simulink model "HX_2023b_mdl"  (R2023b)
settings: Solver=ode4  StartTime=0  StopTime=300  FixedStep=0.01  RelTol=1e-3
undefined symbols (not defined in the file): f11, f22, g11_a, g11_b, g12_a, g21_a, g22_a, g22_b, P0
settings Model: SimulationMode=accelerator  Creator=mohammadodeh  LastModifiedBy=mohammadodeh

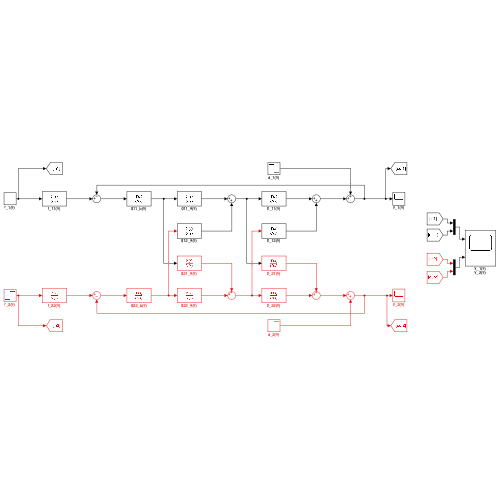
[thumbnail: Simulink's stored preview of the top-level diagram]
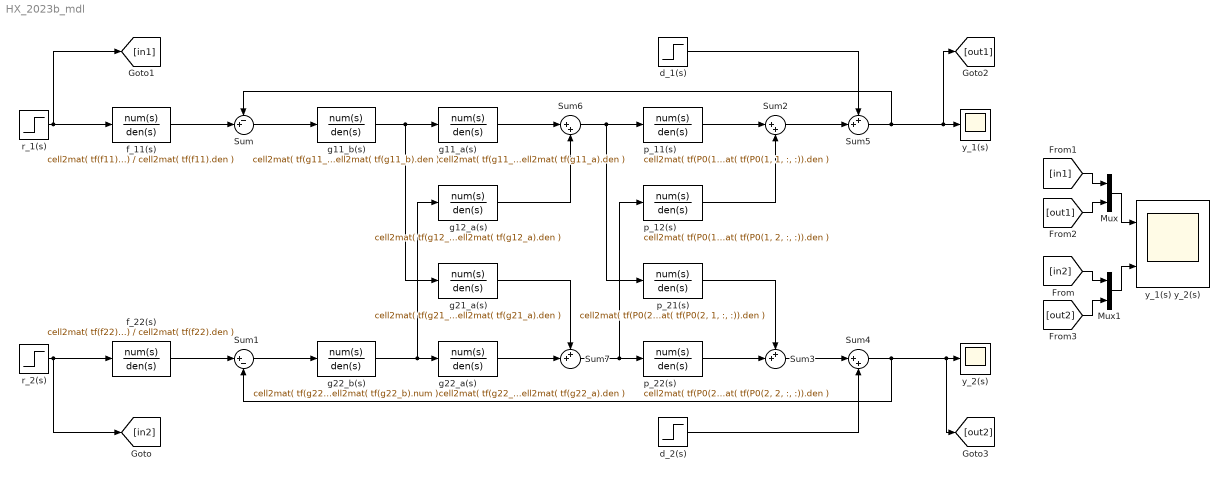
== system HX_2023b_mdl ==
  Mux : Mux  Inputs=2
  Mux1 : Mux  Inputs=2
  Sum : Sum  Inputs=-+|
  Sum1 : Sum  Inputs=|+-
  Sum2 : Sum  Inputs=|++
  Sum3 : Sum  Inputs=++|
  Sum4 : Sum  Inputs=|++
  Sum5 : Sum  Inputs=++|
  Sum6 : Sum  Inputs=|++
  Sum7 : Sum  Inputs=++|
  d_1(s) : Step  Time=250  After=-1  SampleTime=0
  d_2(s) : Step  Time=120  After=0.25  SampleTime=0
  f_11(s) : TransferFcn  Numerator=cell2mat( tf(f11).num )  Denominator=cell2mat( tf(f11).den )
  f_22(s) : TransferFcn  Numerator=cell2mat( tf(f22).num )  Denominator=cell2mat( tf(f22).den )
  g11_a(s) : TransferFcn  Numerator=cell2mat( tf(g11_a).num )  Denominator=cell2mat( tf(g11_a).den )
  g11_b(s) : TransferFcn  Numerator=cell2mat( tf(g11_b).num )  Denominator=cell2mat( tf(g11_b).den )
  g12_a(s) : TransferFcn  Numerator=cell2mat( tf(g12_a).num )  Denominator=cell2mat( tf(g12_a).den )
  g21_a(s) : TransferFcn  Numerator=cell2mat( tf(g21_a).num )  Denominator=cell2mat( tf(g21_a).den )
  g22_a(s) : TransferFcn  Numerator=cell2mat( tf(g22_a).num )  Denominator=cell2mat( tf(g22_a).den )
  g22_b(s) : TransferFcn  Numerator=cell2mat( tf(g22_b).num )  Denominator=cell2mat( tf(g22_b).num )
  p_11(s) : TransferFcn  Numerator=cell2mat( tf(P0(1, 1, :, :)).num )  Denominator=cell2mat( tf(P0(1, 1, :, :)).den )
  p_12(s) : TransferFcn  Numerator=cell2mat( tf(P0(1, 2, :, :)).num )  Denominator=cell2mat( tf(P0(1, 2, :, :)).den )
  p_21(s) : TransferFcn  Numerator=cell2mat( tf(P0(2, 1, :, :)).num )  Denominator=cell2mat( tf(P0(2, 1, :, :)).den )
  p_22(s) : TransferFcn  Numerator=cell2mat( tf(P0(2, 2, :, :)).num )  Denominator=cell2mat( tf(P0(2, 2, :, :)).den )
  r_1(s) : Step  Time=20  SampleTime=0
  r_2(s) : Step  Time=170  SampleTime=0
  y_1(s) : Scope
  y_1(s) y_2(s) : Scope  NumInputPorts=2
  y_2(s) : Scope
  wires:
  f_11(s)/1 -> Sum/2
  Sum/1 -> g11_b(s)/1
  f_22(s)/1 -> Sum1/1
  Sum1/1 -> g22_b(s)/1
  r_1(s)/1 -> [in1], f_11(s)/1
  r_2(s)/1 -> f_22(s)/1, [in2]
  Sum4/1 -> [out2], y_2(s)/1, Sum1/2
  d_1(s)/1 -> Sum5/1
  Sum5/1 -> [out1], y_1(s)/1, Sum/1
  p_21(s)/1 -> Sum3/1
  p_12(s)/1 -> Sum2/2
  d_2(s)/1 -> Sum4/2
  p_22(s)/1 -> Sum3/2
  Sum3/1 -> Sum4/1
  p_11(s)/1 -> Sum2/1
  Sum2/1 -> Sum5/2
  g11_b(s)/1 -> g21_a(s)/1, g11_a(s)/1
  g22_b(s)/1 -> g12_a(s)/1, g22_a(s)/1
  g11_a(s)/1 -> Sum6/1
  Sum6/1 -> p_21(s)/1, p_11(s)/1
  g12_a(s)/1 -> Sum6/2
  g22_a(s)/1 -> Sum7/2
  Sum7/1 -> p_12(s)/1, p_22(s)/1
  g21_a(s)/1 -> Sum7/1
  Mux/1 -> y_1(s) y_2(s)/1
  Mux1/1 -> y_1(s) y_2(s)/2
  [in2] -> Mux1/1
  [in1] -> Mux/1
  [out1] -> Mux/2
  [out2] -> Mux1/2
